simulink model "part3"  (R2018a)
settings: Solver=VariableStepAuto  StartTime=0.0  StopTime=0.1  RelTol=1e-3
libraries: truetime x1
settings Model: Creator=Ismael  LastModifiedBy=Ismael

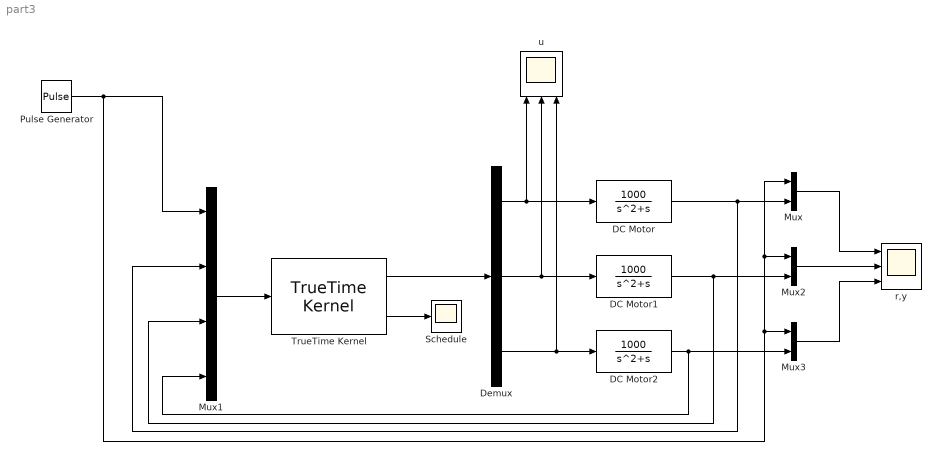
== system part3 ==
  DC Motor : TransferFcn  Numerator=[1000]  Denominator=[1 1 0]
  DC Motor1 : TransferFcn  Numerator=[1000]  Denominator=[1 1 0]
  DC Motor2 : TransferFcn  Numerator=[1000]  Denominator=[1 1 0]
  Demux : Demux  Outputs=3
  Mux : Mux  Inputs=2
  Mux1 : Mux
  Mux2 : Mux  Inputs=2
  Mux3 : Mux  Inputs=2
  "Pulse Generator " : DiscretePulseGenerator  PulseType=Time based  Amplitude=2  Period=1  PulseWidth=50  PhaseDelay=0.1
  Schedule : Scope
  "TrueTime Kernel " : truetime/TrueTime Kernel  sfun=part3_init  args=1  ninputsoutputs=[4 3]  ntriggers=0  trigtype=falling  nwnodenbr=[]  clockoffsetdrift=[0 0]  schedoutput=on  battery=off  poweroutput=off
  r,y : Scope  NumInputPorts=3
  u : Scope  NumInputPorts=3
  wires:
  "TrueTime Kernel "/2 -> Schedule/1
  Mux1/1 -> "TrueTime Kernel "/1
  "Pulse Generator "/1 -> Mux/1, Mux2/1, Mux3/1, Mux1/1
  Demux/1 -> u/1, DC Motor/1
  Demux/2 -> u/2, DC Motor1/1
  Demux/3 -> u/3, DC Motor2/1
  "TrueTime Kernel "/1 -> Demux/1
  Mux2/1 -> r,y/2
  Mux/1 -> r,y/1
  Mux3/1 -> r,y/3
  DC Motor/1 -> Mux1/2, Mux/2
  DC Motor1/1 -> Mux1/3, Mux2/2
  DC Motor2/1 -> Mux1/4, Mux3/2
